simulink model "pid_following"  (R2025a)
settings: Solver=VariableStepAuto  StartTime=0.0  StopTime=10.0  RelTol=1e-3
libraries: mssSimulink x7, simulink_extras x3
settings Model: Creator=SERILEG  LastModifiedBy=SERILEG

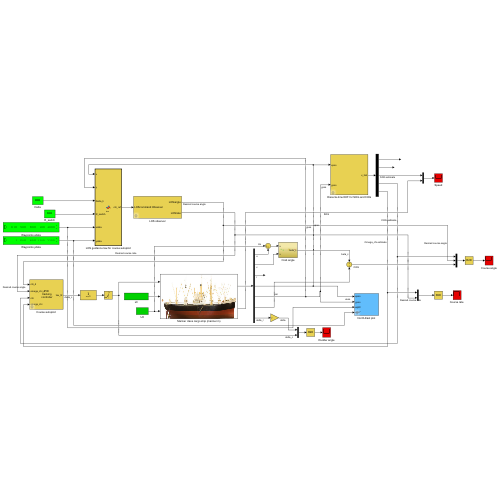
[thumbnail: Simulink's stored preview of the top-level diagram]
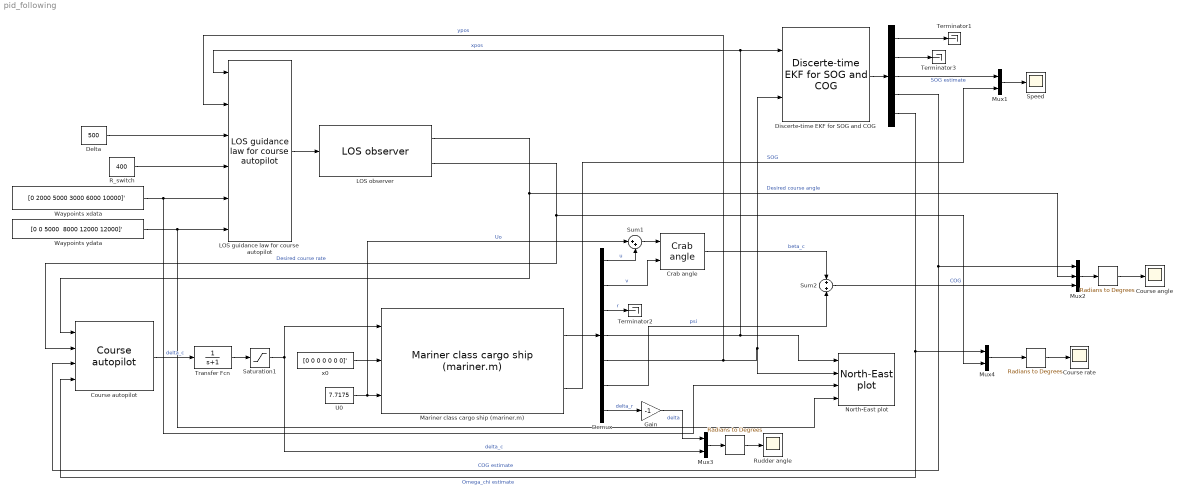
== system pid_following ==
  "  " : simulink_extras/Transformations/Radians to Degrees
  "      " : simulink_extras/Transformations/Radians to Degrees
  "           " : simulink_extras/Transformations/Radians to Degrees
  "            " : Demux  Outputs=5
  Course angle : Scope
      settings: ActiveDisplayYMinimum=-75.71543  ActiveDisplayYMaximum=196.66808  DataLoggingDecimation=10
  "Course autopilot " : mssSimulink/Control/Autopilots/Course autopilot   T_nomoto=107.3  K_nomoto=0.185  Kp=1.45  Td=36.27  Ti=200
  "Course rate " : Scope
      settings: ActiveDisplayYMinimum=-1.22468  ActiveDisplayYMaximum=1.27547  DataLoggingDecimation=10  DataLoggingVariableName=ScopeData3
  Crab angle : mssSimulink/Modelling/Kinematics/Crab angle  SystemSampleTime=-1  VariantActivationTime=update diagram  EmptyChoice=off  PassThrough=off  PassThroughVariantControl=(default)  EmptyChoiceVariantControl=(default)  AllowFlexibleInterface=on  Latency=0  AutoFrameSizeCalculation=off
  Delta : Constant  Value=500
  Demux : Demux  Outputs=7
  Discerte-time EKF for SOG and COG : mssSimulink/Navigation/Estimators/Discerte-time EKF for SOG and COG  alpha_1=0.00001  alpha_2=0.00001  Qd=100*diag([0.1,0.1])  Rd=1000*diag([1 1])  h_samp=0.1
  Gain : Gain  Gain=-1
  LOS guidance law for course autopilot : mssSimulink/Guidance/LOS guidance law for course autopilot  SystemSampleTime=-1  VariantActivationTime=update diagram  EmptyChoice=off  PassThrough=off  PassThroughVariantControl=(default)  EmptyChoiceVariantControl=(default)  AllowFlexibleInterface=on  Latency=0  AutoFrameSizeCalculation=off
  LOS observer : mssSimulink/Guidance/LOS observer  K_f=0.3  alpha=5
  Mariner class cargo ship (mariner.m) : mssSimulink/Marine craft models/Mariner class cargo ship (mariner.m)  SystemSampleTime=-1  VariantActivationTime=update diagram  EmptyChoice=off  PassThrough=off  PassThroughVariantControl=(default)  EmptyChoiceVariantControl=(default)  AllowFlexibleInterface=on  Latency=0  AutoFrameSizeCalculation=off
  Mux1 : Mux  Inputs=2
  Mux2 : Mux  Inputs=3
  Mux3 : Mux  Inputs=2
  Mux4 : Mux  Inputs=2
  North-East plot : mssSimulink/Utilities/Visualization/North-East plot  decimation=10
  R_switch : Constant  Value=400
  Rudder angle : Scope
      settings: ActiveDisplayYMinimum=-50  ActiveDisplayYMaximum=50  DataLoggingDecimation=10
  Saturation1 : Saturate  UpperLimit=40*pi/180  LowerLimit=-40*pi/180
  Speed : Scope
      settings: ActiveDisplayYMinimum=-0.96469  ActiveDisplayYMaximum=8.68219  DataLoggingDecimation=10  DataLoggingVariableName=ScopeData4
  Sum1 : Sum  Inputs=|++
  Sum2 : Sum  Inputs=+|+
  Terminator1 : Terminator
  Terminator2 : Terminator
  Terminator3 : Terminator
  Transfer Fcn : TransferFcn  Denominator=[1 1]
  U0 : Constant  Value=7.7175
  Waypoints xdata : Constant  Value=[0 2000 5000 3000 6000 10000]'
  Waypoints ydata : Constant  Value="[0 0 5000  8000 12000 12000]'"
  x0 : Constant  Value=[0 0 0 0 0 0 0]'
  wires:
  Delta/1 -> LOS guidance law for course autopilot/3
  Mux1/1 -> Speed/1
  Waypoints ydata/1 -> LOS guidance law for course autopilot/6, North-East plot/4
  U0/1 -> Sum1/1, Mariner class cargo ship (mariner.m)/3  "Uo"
  "      "/1 -> Rudder angle/1
  Crab angle/1 -> Sum2/1  "beta_c"
  "            "/2 -> Terminator3/1
  Discerte-time EKF for SOG and COG/1 -> "            "/1
  Waypoints xdata/1 -> LOS guidance law for course autopilot/5, North-East plot/3
  Mux4/1 -> "  "/1
  Demux/3 -> Terminator2/1  "r"
  "            "/1 -> Terminator1/1
  Sum1/1 -> Crab angle/1
  "  "/1 -> "Course rate "/1
  LOS observer/1 -> "Course autopilot "/1, Mux2/2  "Desired course angle"
  Mariner class cargo ship (mariner.m)/1 -> Demux/1
  Saturation1/1 -> Mux3/2, Mariner class cargo ship (mariner.m)/1  "delta_c"
  R_switch/1 -> LOS guidance law for course autopilot/4
  Demux/5 -> LOS guidance law for course autopilot/2, Discerte-time EKF for SOG and COG/2, North-East plot/2  "ypos"
  Demux/6 -> Sum2/2  "psi"
  Gain/1 -> Mux3/1  "delta"
  Transfer Fcn/1 -> Saturation1/1
  x0/1 -> Mariner class cargo ship (mariner.m)/2
  LOS guidance law for course autopilot/1 -> LOS observer/1
  LOS observer/2 -> "Course autopilot "/2, Mux4/2  "Desired course rate"
  Mariner class cargo ship (mariner.m)/2 -> Mux1/2  "SOG"
  "            "/5 -> "Course autopilot "/4, Mux4/1  "Omega_chi estimate"
  "Course autopilot "/1 -> Transfer Fcn/1  "delta_c"
  "            "/3 -> Mux1/1  "SOG estimate"
  Demux/2 -> Crab angle/2  "v"
  Demux/4 -> North-East plot/1, Discerte-time EKF for SOG and COG/1, LOS guidance law for course autopilot/1  "xpos"
  "           "/1 -> Course angle/1
  Demux/1 -> Sum1/2  "u"
  Sum2/1 -> Mux2/3  "COG"
  Mux2/1 -> "           "/1
  Mux3/1 -> "      "/1
  Demux/7 -> Gain/1  "delta_r"
  "            "/4 -> "Course autopilot "/3, Mux2/1  "COG estimate"
